simulink subsystem "pdplus_control_ref_subsys"  (R2022b)
settings: Solver=VariableStepAuto  StartTime=0.0  StopTime=10.0  RelTol=1e-3
undefined symbols (not defined in the file): ctrl_param, param_robot
settings Model: Creator=emu  LastModifiedBy=rslstudent

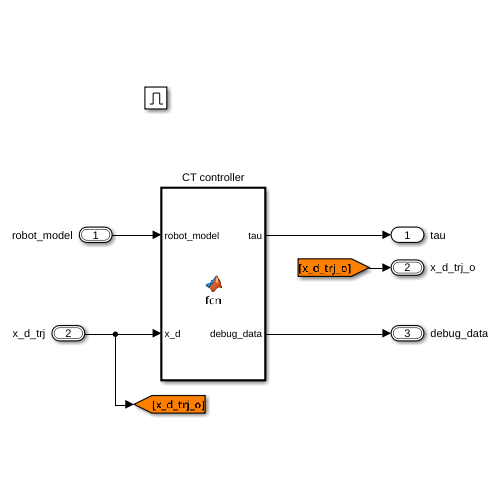
[thumbnail: Simulink's stored preview of the top-level diagram]
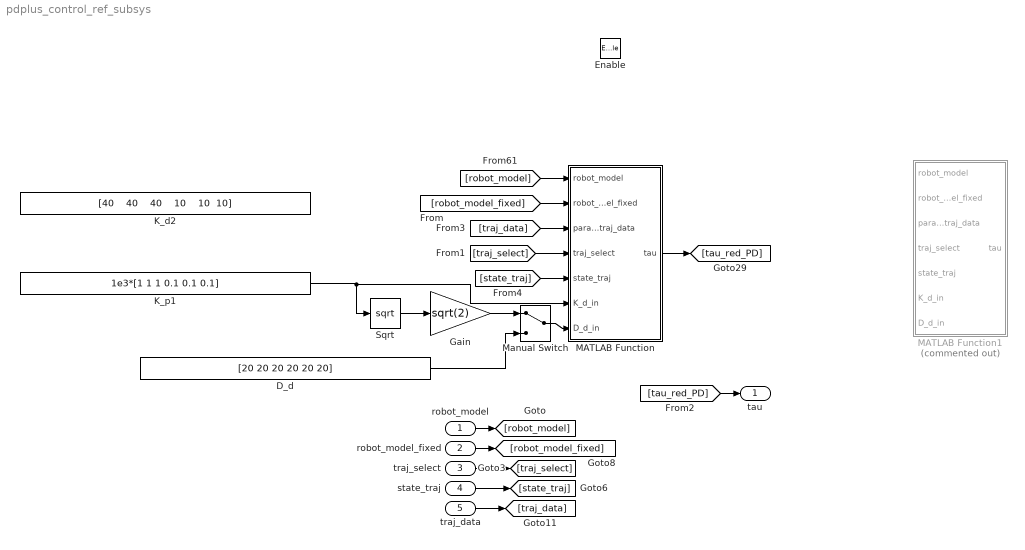
== system pdplus_control_ref_subsys ==
  robot_model : Inport  OutDataTypeStr=Bus: robot_model
  robot_model_fixed : Inport  Port=2  OutDataTypeStr=Bus: robot_model
  traj_select : Inport  Port=3
  state_traj : Inport  Port=4  OutDataTypeStr=Bus: state_traj_bus
  traj_data : Inport  Port=5  OutDataTypeStr=Bus: traj_data_bus
  Enable : EnablePort
  D_d : Constant  Value=[20 20 20 20 20 20]
  Gain : Gain  Gain=sqrt(2)
  K_d2 : Constant  Value="[40    40    40    10    10  10]"
  K_p1 : Constant  Value=1e3*[1 1 1 0.1 0.1 0.1]
  MATLAB Function : MATLAB Function  TreatAsAtomicUnit=on
  MATLAB Function1 : MATLAB Function  Commented=on  TreatAsAtomicUnit=on
  Manual Switch : ManualSwitch
  Sqrt : Sqrt
  tau : Outport
  wires:
  [state_traj] -> MATLAB Function/5(state_traj)
  state_traj/1 -> [state_traj]
  [traj_select] -> MATLAB Function/4(traj_select)
  traj_select/1 -> [traj_select]
  [traj_data] -> MATLAB Function/3(param_traj_data)
  traj_data/1 -> [traj_data]
  D_d/1 -> Manual Switch/2
  Gain/1 -> Manual Switch/1
  Manual Switch/1 -> MATLAB Function/7(D_d_in)
  K_p1/1 -> MATLAB Function/6(K_d_in), Sqrt/1
  Sqrt/1 -> Gain/1
  [robot_model] -> MATLAB Function/1(robot_model)
  robot_model/1 -> [robot_model]
  MATLAB Function/1(tau) -> [tau_red_PD]
  [tau_red_PD] -> tau/1
  robot_model_fixed/1 -> [robot_model_fixed]
  [robot_model_fixed] -> MATLAB Function/2(robot_model_fixed)

== matlab function pdplus_control_ref_subsys/MATLAB Function ==
  data: robot_model input Bus: robot_model; robot_model_fixed input Bus: robot_model; tau output; param_traj_data input Bus: traj_data_bus; traj_select input; state_traj input Bus: state_traj_bus; K_d_in input; D_d_in input; ctrl_param parameter; param_robot parameter
function tau  = fcn(robot_model, robot_model_fixed, param_traj_data, traj_select, state_traj, K_d_in, D_d_in, ctrl_param, param_robot)

persistent cnt;
persistent run_flag;

if(isempty(cnt))
    cnt = 1;
    run_flag = 0;
end

% Parameters
%q = robot_model.q;      % generalized coordinates
q_p = robot_model.q_p;  % time derivative of generalized coordinates

M = robot_model.M;      % inertia matrix
C = robot_model.C;      % coriolis matrix
%g = robot_model.g;      % gravitational forces
%C_rnea = robot_model.C_rnea; % C_rnea(q, q_p) = C(q, q_p)q_p + g(q) = n(q, q_p)

J = robot_model.J;      % geometric jacobian to end-effector

J_p = robot_model.J_p;  % time derivative of geometric jacobian to end-effector
H = robot_model.H;

n = param_robot.n_DOF;
n_red = param_robot.n_red;
n_indices = param_robot.n_indices;
n_indices_fixed = param_robot.n_indices_fixed;

yt_indices = param_robot.yt_indices;
yr_indices = param_robot.yr_indices;
y_indices =  [yt_indices 3+yr_indices];

m = numel(yt_indices) + numel(yr_indices);

M_red = M(n_indices, n_indices);
C_red = C(n_indices, n_indices);
%C_rnea_red = C_rnea(n_indices);

J_red = J(y_indices, n_indices);
J_p_red = J_p(y_indices, n_indices);

%g_red = g(n_indices);

% Control parameters
%D_d = ctrl_param.pd.D_d(y_indices, y_indices);
%K_d = ctrl_param.pd.K_d(y_indices, y_indices);
D_d = diag(D_d_in(y_indices));
K_d = diag(K_d_in(y_indices));

% Current Pose of Endeffector
x_p = J*q_p;

p = H(yt_indices,4);
R = H(1:3,1:3);
p_p  = x_p(yt_indices);
omega_e = x_p(3+yr_indices); % Drehwinkelgeschwindigkeit des Endeffektors

% Desired Trajectory
p_d    = param_traj_data.p_d(yt_indices, cnt, traj_select);
p_d_p  = param_traj_data.p_d_p(yt_indices, cnt, traj_select);
p_d_pp = param_traj_data.p_d_pp(yt_indices, cnt, traj_select);

q_d = param_traj_data.q_d(:, cnt, traj_select);
R_d = param_traj_data.R_d(:, :, cnt, traj_select);
omega_d = param_traj_data.omega_d(yr_indices, cnt, traj_select);
omega_d_p = param_traj_data.omega_d_p(yr_indices, cnt, traj_select);

% Errors
%RR = R*R_d';
%RR = R_d'*R;
%q_err_tmp   = rotm2quat_v4(RR);
quat = rotm2quat_v4(R);
quat = quat * my_sign(quat(1));
q_d = q_d * my_sign(q_d(1));
q_err_tmp = quat_mult(quat, quat_inv(q_d));
%RR = R*R_d' - R_d*R';
%q_err_tmp = [1; RR(3,2); RR(1,3); RR(2,1)];

q_err = q_err_tmp(1+yr_indices);

x_err   = [p-p_d;      q_err];   % Error as quaternion
x_err_p = [p_p-p_d_p;  omega_e-omega_d];
x_d_p   = [p_d_p;      omega_d];
x_d_pp  = [p_d_pp;     omega_d_p];


% CT control law
%% Cartesian Endeffector Pose

sing_method = ctrl_param.regularization.mode;
j = [];

if(sing_method == 0)
    J_pinv = J_red\eye(m);
elseif(sing_method == 1) % add +k*E
    k = ctrl_param.regularization.k;
    J_pinv = (J_red'*J_red + k*eye(n_red))\J_red';
elseif(sing_method == 2) % add +lambda*E
    W_bar_N = ctrl_param.regularization.W_bar_N(n_indices);
    W_E = ctrl_param.regularization.W_E(y_indices, y_indices);

    e = x_err;
    E_k = 1/2 * e' * W_E * e;
    W_N = eye(n_red)*E_k + W_bar_N;

    [~, S, V] = svd(sqrt(W_E)*J_red);

    S_nonzero = diag(diag(S)); % get only nonzero sing values

    H_k = V*(S_nonzero^2)*V' + W_N;
    J_pinv = H_k\J_red';
elseif(sing_method == 3 || sing_method == 4 || sing_method == 5) % remove small singular values
    % Perform SVD
    [U, S, V] = svd(J_red);
    
    % Set a threshold for small singular values
    epsilon = ctrl_param.regularization.eps; % Adjust epsilon as needed
    
    if(sing_method == 3)
        % Threshold small singular values in S
        S_new = diag(max(diag(S), epsilon));  % Creates a diagonal matrix with thresholded values
        S(1:n_red, 1:n_red) = S_new;
    elseif(sing_method == 4)
        idx = diag(S) < epsilon;
        S(idx, idx) = sqrt(S(idx, idx)^2 + eye(sum(idx)) * epsilon^2);
    else%if(sing_method == 5)
        sigma_arr = diag(S);
        idx = sigma_arr < epsilon;
        sign_sigma = 2*(sigma_arr(idx) >= 0) - 1;
        S(idx, idx) = sign_sigma / max(param_robot.q_limit_upper);
    end
    
    % Reconstruct the matrix with modified singular values
    J_new = U * S * V';
    J_pinv = pinv(J_new);
elseif(sing_method == 6) % collinearity   
    if(rank(J_red, 1e-1) < m)
        J_tilde = J_red./vecnorm(J_red);
        JJ_colin = J_tilde'*J_tilde;
        [i,j] = find(abs(tril(JJ_colin) - eye(n_red)) > ctrl_param.regularization.eps_collinear);

        J_red(:, j) = 0;
        
        J_pinv = pinv(J_red);
    else
        J_pinv = J_red\eye(m);
    end
else%if(sing_method == 7) % nach Steinboeck Optreg
    J_scale = 1./vecnorm(J_red);
    J_tilde = J_red.*J_scale;
    JJ_colin = J_tilde'*J_tilde;
    %[V, D] = eig(JJ_colin);

    [U, D, V] = svd(JJ_colin);

    V_new = real(V(:, real(diag(D)) > ctrl_param.regularization.lambda_min));

    T_bar = J_scale' .* V_new;

    J_new = J_red*T_bar;

    J_pinv = T_bar * (J_new \ eye(m));
end

J_pinv_T = J_pinv';
Lambda = J_pinv_T*M_red*J_pinv;
Lambda = 1/2 * (Lambda + Lambda');
mu = J_pinv_T*(C_red - M_red*J_pinv*J_p_red)*J_pinv;
%mu = Lambda * (J / (M) * C - J_p);
%F_g = J_pinv_T*g_red; gravity is ignored here!

%Lambda = inv(J)' * (C - M * inv(J)*J_p)*inv(J);
%mu = inv(J)' * (C - M*inv(J)*J_p)*inv(J);
%F_g = inv(J)'*g;

F_red = Lambda*x_d_pp + mu*x_d_p - D_d*x_err_p - K_d*x_err;

tau_red = J_red' * F_red;

q_pp_red = M_red\(tau_red - C(n_indices, :)*q_p - 0); % gravity is ignored here
q_pp = zeros(n, 1);
q_pp(n_indices) = q_pp_red;

% v1
%tau = M*q_pp + C*q_p;

%v2
tau = zeros(n,1);
tau(n_indices) = tau_red;

% e_fixed = zeros(n,1);
% e_fixed(n_indices_fixed)=1;
% K = eye(n);
% K(:,n_indices_fixed) = [];
% 
% tau(n_indices_fixed) = e_fixed' * (M*K*q_pp_red + C*q_p);
%v3: fehler zw. v2,v3 zu v1: 1e-16
tau(n_indices_fixed) = M(n_indices_fixed,:)*q_pp + C(n_indices_fixed,:)*q_p;

[run_flag, cnt] = update_traj_cnt(state_traj, run_flag, cnt, param_traj_data.N);

end

function y = my_sign(x)
    y = (x >= 0)*2 - 1;
end

== matlab function pdplus_control_ref_subsys/MATLAB Function1 ==
  data: robot_model input Bus: robot_model; robot_model_fixed input Bus: robot_model; tau output; param_traj_data input Bus: traj_data_bus; traj_select input; state_traj input Bus: state_traj_bus; K_d_in input; D_d_in input; ctrl_param parameter; param_robot parameter
function tau  = fcn(robot_model, robot_model_fixed, param_traj_data, traj_select, state_traj, K_d_in, D_d_in, ctrl_param, param_robot)

persistent cnt;
persistent run_flag;

if(isempty(cnt))
    cnt = 1;
    run_flag = 0;
end

% Parameters
%q = robot_model.q;      % generalized coordinates
q_p = robot_model.q_p;  % time derivative of generalized coordinates

M = robot_model.M;      % inertia matrix
C = robot_model.C;      % coriolis matrix
%g = robot_model.g;      % gravitational forces
%C_rnea = robot_model.C_rnea; % C_rnea(q, q_p) = C(q, q_p)q_p + g(q) = n(q, q_p)

%J = robot_model.J;      % geometric jacobian to end-effector

%J_p = robot_model.J_p;  % time derivative of geometric jacobian to end-effector
%H = robot_model.H;

n = param_robot.n_DOF;
n_red = param_robot.n_red;
n_indices = param_robot.n_indices;
n_indices_fixed = param_robot.n_indices_fixed;

yt_indices = param_robot.yt_indices;
yr_indices = param_robot.yr_indices;
y_indices =  [yt_indices 3+yr_indices];

m = numel(yt_indices) + numel(yr_indices);

q_fixed = robot_model_fixed.q;
q_p_fixed = robot_model_fixed.q_p;
H_red = robot_model_fixed.H;
M_fixed = robot_model_fixed.M;
C_fixed = robot_model_fixed.C;
J_fixed = robot_model_fixed.J;
J_p_fixed = robot_model_fixed.J_p;

q_red = q_fixed(n_indices);
q_p_red = q_p_fixed(n_indices);

M_red = M_fixed(n_indices, n_indices);
C_red = C_fixed(n_indices, n_indices);

J_red = J_fixed(y_indices, n_indices);
J_p_red = J_p_fixed(y_indices, n_indices);

%g_red = g(n_indices);

% Control parameters
%D_d = ctrl_param.pd.D_d(y_indices, y_indices);
%K_d = ctrl_param.pd.K_d(y_indices, y_indices);
D_d = diag(D_d_in(y_indices));
K_d = diag(K_d_in(y_indices));

% Current Pose of Endeffector
x_p = J_red*q_red;

p = H_red(yt_indices,4);
R = H_red(1:3,1:3);
p_p  = x_p(yt_indices);
omega_e = x_p(3+yr_indices); % Drehwinkelgeschwindigkeit des Endeffektors

% Desired Trajectory
p_d    = param_traj_data.p_d(yt_indices, cnt, traj_select);
p_d_p  = param_traj_data.p_d_p(yt_indices, cnt, traj_select);
p_d_pp = param_traj_data.p_d_pp(yt_indices, cnt, traj_select);

R_d = param_traj_data.R_d(:, :, cnt, traj_select);
omega_d = param_traj_data.omega_d(yr_indices, cnt, traj_select);
omega_d_p = param_traj_data.omega_d_p(yr_indices, cnt, traj_select);

% Errors
RR = R'*R_d;
%RR = R_d*R';
q_err_tmp   = rotm2quat_v4(RR);
%RR = R*R_d' - R_d*R';
%q_err_tmp = [1; RR(3,2); RR(1,3); RR(2,1)];

q_err = q_err_tmp(1+yr_indices);
%q_err = q_err * my_sign(q_err(1));

x_err   = [p-p_d;      q_err];   % Error as quaternion
x_err_p = [p_p-p_d_p;  omega_e-omega_d];
x_d_p   = [p_d_p;      omega_d];
x_d_pp  = [p_d_pp;     omega_d_p];


% CT control law
%% Cartesian Endeffector Pose

sing_method = ctrl_param.regularization.mode;
j = [];

if(sing_method == 0)
    J_pinv = J_red\eye(m);
elseif(sing_method == 1) % add +k*E
    k = ctrl_param.regularization.k;
    J_pinv = (J_red'*J_red + k*eye(n_red))\J_red';
elseif(sing_method == 2) % add +lambda*E
    W_bar_N = ctrl_param.regularization.W_bar_N(n_indices);
    W_E = ctrl_param.regularization.W_E(y_indices, y_indices);

    e = x_err;
    E_k = 1/2 * e' * W_E * e;
    W_N = eye(n_red)*E_k + W_bar_N;

    [~, S, V] = svd(sqrt(W_E)*J_red);

    S_nonzero = diag(diag(S)); % get only nonzero sing values

    H_k = V*(S_nonzero^2)*V' + W_N;
    J_pinv = H_k\J_red';
elseif(sing_method == 3 || sing_method == 4 || sing_method == 5) % remove small singular values
    % Perform SVD
    [U, S, V] = svd(J_red);
    
    % Set a threshold for small singular values
    epsilon = ctrl_param.regularization.eps; % Adjust epsilon as needed
    
    if(sing_method == 3)
        % Threshold small singular values in S
        S_new = diag(max(diag(S), epsilon));  % Creates a diagonal matrix with thresholded values
        S(1:n_red, 1:n_red) = S_new;
    elseif(sing_method == 4)
        idx = diag(S) < epsilon;
        S(idx, idx) = sqrt(S(idx, idx)^2 + eye(sum(idx)) * epsilon^2);
    else%if(sing_method == 5)
        sigma_arr = diag(S);
        idx = sigma_arr < epsilon;
        sign_sigma = 2*(sigma_arr(idx) >= 0) - 1;
        S(idx, idx) = sign_sigma / max(param_robot.q_limit_upper);
    end
    
    % Reconstruct the matrix with modified singular values
    J_new = U * S * V';
    J_pinv = pinv(J_new);
elseif(sing_method == 6) % collinearity   
    if(rank(J_red, 1e-1) < m)
        J_tilde = J_red./vecnorm(J_red);
        JJ_colin = J_tilde'*J_tilde;
        [i,j] = find(abs(tril(JJ_colin) - eye(n_red)) > ctrl_param.regularization.eps_collinear);

        J_red(:, j) = 0;
        
        J_pinv = pinv(J_red);
    else
        J_pinv = J_red\eye(m);
    end
else%if(sing_method == 7) % nach Steinboeck Optreg
    J_scale = 1./vecnorm(J_red);
    J_tilde = J_red.*J_scale;
    JJ_colin = J_tilde'*J_tilde;
    %[V, D] = eig(JJ_colin);

    [U, D, V] = svd(JJ_colin);

    V_new = real(V(:, real(diag(D)) > ctrl_param.regularization.lambda_min));

    T_bar = J_scale' .* V_new;

    J_new = J_red*T_bar;

    J_pinv = T_bar * (J_new \ eye(m));
end

J_pinv_T = J_pinv';
Lambda = J_pinv_T*M_red*J_pinv;
Lambda = 1/2 * (Lambda + Lambda');
mu = J_pinv_T*(C_red - M_red*J_pinv*J_p_red)*J_pinv;
%mu = Lambda * (J / (M) * C - J_p);
%F_g = J_pinv_T*g_red; gravity is ignored here!

%Lambda = inv(J)' * (C - M * inv(J)*J_p)*inv(J);
%mu = inv(J)' * (C - M*inv(J)*J_p)*inv(J);
%F_g = inv(J)'*g;

F_red = Lambda*x_d_pp + mu*x_d_p - D_d*x_err_p - K_d*x_err;

tau_red = J_red' * F_red;

q_pp_red = M(n_indices,n_indices)\(tau_red - C(n_indices, :)*q_p - 0); % gravity is ignored here
%q_pp_red = M_red\(tau_red - C_red*q_p_red - 0); % gravity is ignored here
q_pp = zeros(n, 1);
q_pp(n_indices) = q_pp_red;

% v1
%tau = M*q_pp + C*q_p;

%v2 fehler zw. v2 zu v1: 1e-16
tau = zeros(n,1);
tau(n_indices) = tau_red;
tau(n_indices_fixed) = M(n_indices_fixed,:)*q_pp + C(n_indices_fixed,:)*q_p;

%disp(tau(n_indices) - tau_red)

[run_flag, cnt] = update_traj_cnt(state_traj, run_flag, cnt, param_traj_data.N);

end

function y = my_sign(x)
    y = (x >= 0)*2 - 1;
end
